simulink model "LAB6_TELEMETRY"  (R2024a)
settings: Solver=FixedStepAuto  StartTime=0.0  StopTime=1000  FixedStep=1e-3  RelTol=1e-3
libraries: instrumentseriallib x2
settings Model: Creator=User  LastModifiedBy=anton
settings ModelReferenceCC: EnableRefExpFcnMdlSchedulingChecks=on
settings RTWCC: GPUComputeCapability=3.5

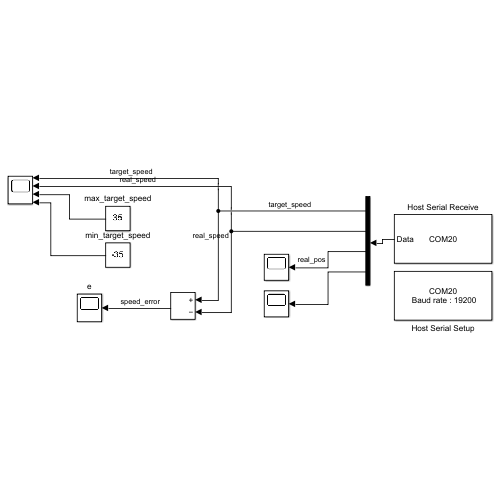
[thumbnail: Simulink's stored preview of the top-level diagram]
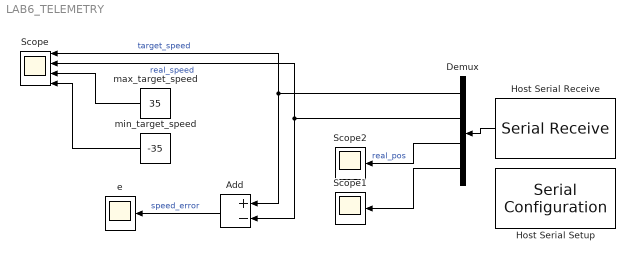
== system LAB6_TELEMETRY ==
  Add : Sum  Inputs=+-
  Demux : Demux
  Host Serial Receive : instrumentseriallib/Serial Receive  PortSel=COM20  Port=COM20  ComPort=COM20  DataType=single  SaveDataType=uint8  ToggleHeader=on  Header='N'  ToggleDataSize=on  DataSize=4  ToggleTerminator=on  Terminator=Custom terminator  CustomTerminator='E'  InputFormat=Column major  EnableBlockingMode=on  ActionDataUnavailable=Output last received value  ActionWhenDataUnavailable=Output last received value  CustomValue=0  SampleTime=0.1  SimulateUsing=Interpreted execution  BlockInModel=on  aMode=5
      settings: LibrarySourceBlock=mcblib/Protection and Diagnostics/Host Serial Receive
  Host Serial Setup : instrumentseriallib/Serial Configuration  Priority=-99  PortSel=COM20  Port=COM20  ComPort=COM20  BaudRate=19200  DataBits=8  Parity=none  StopBits=1  ByteOrder=little-endian  FlowControl=none  Timeout=1.0  SimulateUsing=Interpreted execution  BlockInModel=on  aMode=5
      settings: LibrarySourceBlock=mcblib/Protection and Diagnostics/Host Serial Setup
  Scope : Scope  NumInputPorts=4
  Scope1 : Scope
  Scope2 : Scope
  e : Scope
  max_target_speed : Constant  Value=35
  min_target_speed : Constant  Value=-35
  wires:
  Host Serial Receive/1 -> Demux/1
  Demux/1 -> Scope/1, Add/1  "target_speed"
  Demux/2 -> Add/2, Scope/2  "real_speed"
  Demux/3 -> Scope2/1  "real_pos"
  Add/1 -> e/1  "speed_error"
  max_target_speed/1 -> Scope/3
  min_target_speed/1 -> Scope/4
  Demux/4 -> Scope1/1
